simulink model "simulation_DICBF_"  (R2022a)
settings: Solver=VariableStepAuto  StartTime=0.0  StopTime=simTime  FixedStep=0.01  RelTol=1e-3
values from neighbouring files (symbols this model uses):
  Kd = 1    [setup.m]    (also in setup_DICBF.m)
  Kp = 0.2    [setup.m]    (also in setup_DICBF.m)
  M = 1*eye(2)    [setup.m]    (also in setup_DICBF.m)
  M2 = M    [setup_DICBF.m]
  mu = 1    [setup.m]    (also in setup_DICBF.m = 0.8)
  obstacles = setup_environment(MAP)    [setup_DICBF.m]
  qdotstart = [0,0]    [setup.m]    (also in setup_DICBF.m = [0 ; 0])
  qg = [4, -1]    [setup.m]    (also in setup_DICBF.m)
  qstart = [0,0]    [setup.m]    (also in setup_DICBF.m = [0 ; 0])
  threshold_skip = 0.0    (= 0)    [setup.m]    (also in setup_DICBF.m = 0.1)
libraries: slctrlblks x1
settings Model: Creator=mirkomizzoni  LastModifiedBy=dennis

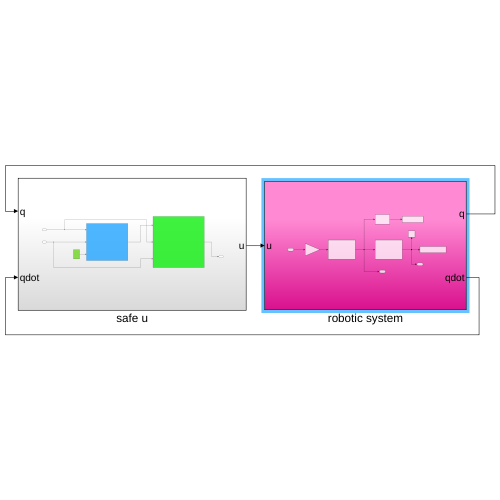
[thumbnail: Simulink's stored preview of the top-level diagram]
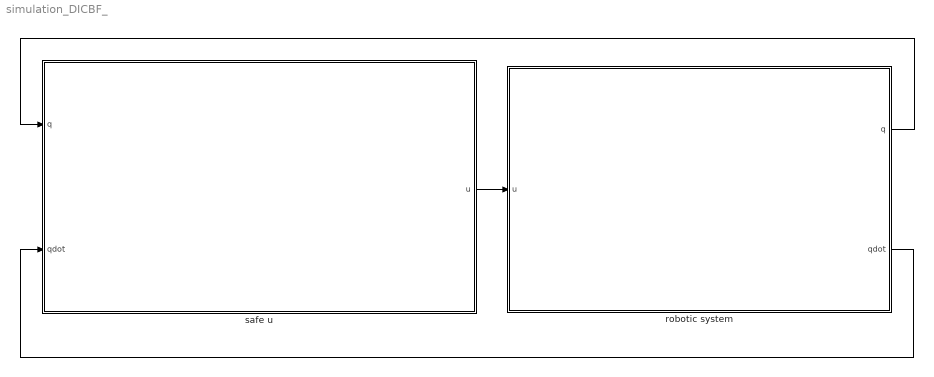
== system simulation_DICBF_ ==
  robotic system : Subsystem
  safe u : Subsystem
  wires:
  safe u/1(u) -> robotic system/1(u)
  robotic system/1(q) -> safe u/1(q)
  robotic system/2(qdot) -> safe u/2(qdot)

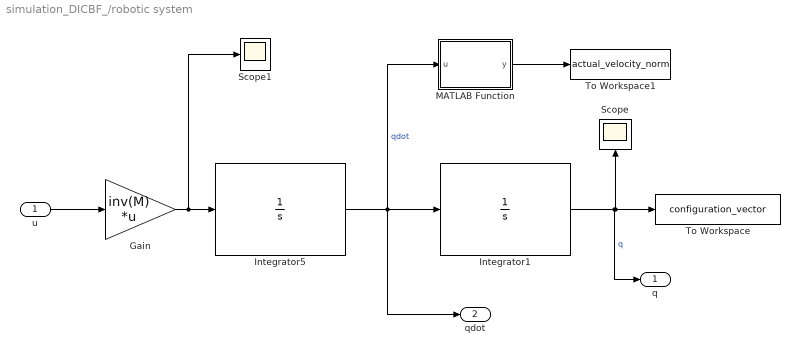
== system simulation_DICBF_/robotic system ==
  u : Inport
  Gain : Gain  Gain=inv(M)  Multiplication=Matrix(K*u)
  Integrator1 : Integrator  InitialCondition=qstart
  Integrator5 : Integrator  InitialCondition=qdotstart
  MATLAB Function : MATLAB Function  TreatAsAtomicUnit=on
  Scope : Scope
  Scope1 : Scope
  To Workspace : ToWorkspace  VariableName=configuration_vector  SaveFormat=Timeseries  SampleTime=0.01
  To Workspace1 : ToWorkspace  VariableName=actual_velocity_norm  SaveFormat=Timeseries  SampleTime=0.01
  q : Outport
  qdot : Outport  Port=2
  wires:
  Integrator5/1 -> qdot/1, MATLAB Function/1(u), Integrator1/1  "qdot"
  Integrator1/1 -> To Workspace/1, Scope/1, q/1  "q"
  MATLAB Function/1(y) -> To Workspace1/1
  Gain/1 -> Scope1/1, Integrator5/1
  u/1 -> Gain/1

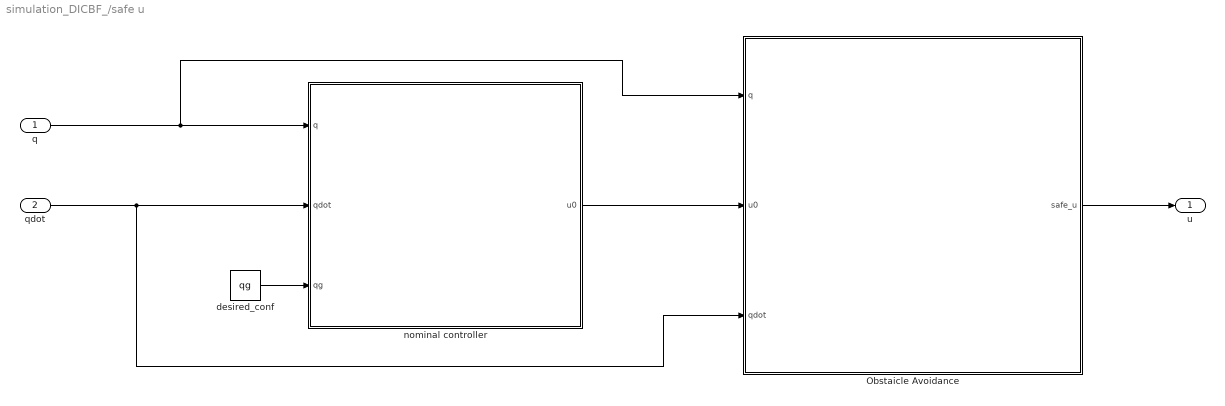
== system simulation_DICBF_/safe u ==
  q : Inport
  qdot : Inport  Port=2
  Obstaicle Avoidance : Subsystem
  desired_conf : Constant  Value=qg
  nominal controller : Subsystem
  u : Outport
  wires:
  desired_conf/1 -> nominal controller/3(qg)
  nominal controller/1(u0) -> Obstaicle Avoidance/2(u0)
  Obstaicle Avoidance/1(safe_u) -> u/1
  q/1 -> Obstaicle Avoidance/1(q), nominal controller/1(q)
  qdot/1 -> Obstaicle Avoidance/3(qdot), nominal controller/2(qdot)

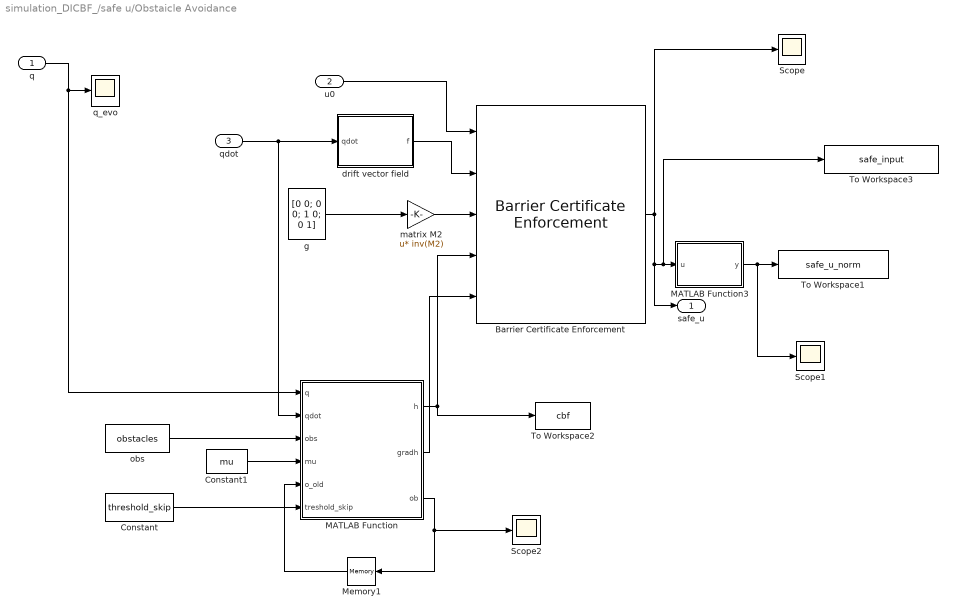
== system simulation_DICBF_/safe u/Obstaicle Avoidance ==
  q : Inport
  u0 : Inport  Port=2
  qdot : Inport  Port=3
  Barrier Certificate Enforcement : slctrlblks/Barrier Certificate Enforcement  nx=4  nu=2  nc=1  gamma=alpha  beta=1  external_umax=off  external_umin=off  Ts=0.01  maxiter=200  tol=1e-06  output_exitflag=off
      settings: SourceProductBaseCode=SD
  Constant : Constant  Value=threshold_skip
  Constant1 : Constant  Value=mu
  MATLAB Function : MATLAB Function  TreatAsAtomicUnit=on
  MATLAB Function3 : MATLAB Function  TreatAsAtomicUnit=on
  Memory1 : Memory  InitialCondition=obstacles(:,1);
  Scope : Scope
  Scope1 : Scope
  Scope2 : Scope
  To Workspace1 : ToWorkspace  VariableName=safe_u_norm  SaveFormat=Timeseries  SampleTime=0.01
  To Workspace2 : ToWorkspace  VariableName=cbf  SaveFormat=Timeseries  SampleTime=0.01
  To Workspace3 : ToWorkspace  VariableName=safe_input  SaveFormat=Timeseries  SampleTime=0.01
  drift vector field : MATLAB Function  TreatAsAtomicUnit=on
  g : Constant  Value=[0 0; 0 0; 1 0; 0 1]  VectorParams1D=off
  matrix M2 : Gain  Gain=inv(M2)  Multiplication=Matrix(u*K)
  obs : Constant  Value=obstacles  VectorParams1D=off
  q_evo : Scope
  safe_u : Outport
  wires:
  q/1 -> MATLAB Function/1(q), q_evo/1
  qdot/1 -> MATLAB Function/2(qdot), drift vector field/1(qdot)
  MATLAB Function3/1(y) -> Scope1/1, To Workspace1/1
  u0/1 -> Barrier Certificate Enforcement/1
  drift vector field/1(f) -> Barrier Certificate Enforcement/2
  Barrier Certificate Enforcement/1 -> To Workspace3/1, MATLAB Function3/1(u), safe_u/1, Scope/1
  g/1 -> matrix M2/1
  matrix M2/1 -> Barrier Certificate Enforcement/3
  MATLAB Function/1(h) -> Barrier Certificate Enforcement/4, To Workspace2/1
  Constant1/1 -> MATLAB Function/4(mu)
  obs/1 -> MATLAB Function/3(obs)
  Constant/1 -> MATLAB Function/6(treshold_skip)
  MATLAB Function/2(gradh) -> Barrier Certificate Enforcement/5
  MATLAB Function/3(ob) -> Scope2/1, Memory1/1
  Memory1/1 -> MATLAB Function/5(o_old)

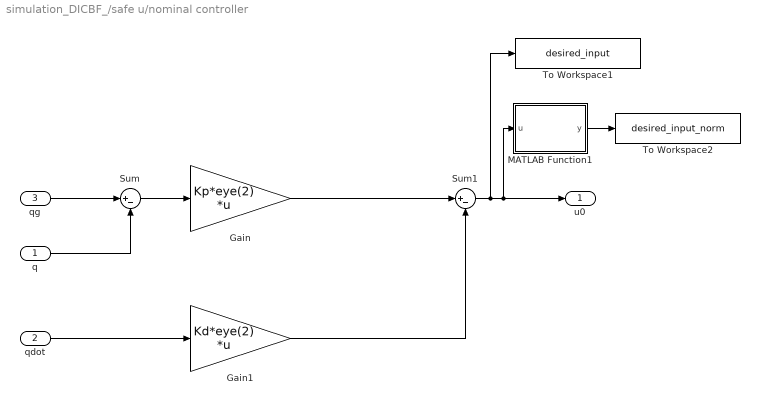
== system simulation_DICBF_/safe u/nominal controller ==
  q : Inport
  qdot : Inport  Port=2
  qg : Inport  Port=3
  Gain : Gain  Gain=Kp*eye(2)  Multiplication=Matrix(K*u)
  Gain1 : Gain  Gain=Kd*eye(2)  Multiplication=Matrix(K*u)
  MATLAB Function1 : MATLAB Function  TreatAsAtomicUnit=on
  Sum : Sum  Inputs=|+-
  Sum1 : Sum  Inputs=|+-
  To Workspace1 : ToWorkspace  VariableName=desired_input  SaveFormat=Timeseries  SampleTime=0.01
  To Workspace2 : ToWorkspace  VariableName=desired_input_norm  SaveFormat=Timeseries  SampleTime=0.01
  u0 : Outport
  wires:
  MATLAB Function1/1(y) -> To Workspace2/1
  q/1 -> Sum/2
  qg/1 -> Sum/1
  Sum/1 -> Gain/1
  Gain/1 -> Sum1/1
  qdot/1 -> Gain1/1
  Gain1/1 -> Sum1/2
  Sum1/1 -> To Workspace1/1, MATLAB Function1/1(u), u0/1

== matlab function simulation_DICBF_/safe u/Obstaicle Avoidance/MATLAB Function ==
  data: q input; qdot input; obs input; h output; gradh output; mu input; o_old input; treshold_skip input; ob output
function [h, gradh, ob]= compute_h_gradh(q, qdot, obs, mu, o_old, treshold_skip)
    [~,n] = size(obs);
    o1 = obs(:,1);
    h = first_part_h(q,o1)+second_part_h(o1(1:2),q,qdot,mu);
    gradh = gradient(o1(1:2),q, mu, qdot);
    ob = o1;
    for i=2:n
        oi = obs(:,i);
        t = first_part_h(q,oi)+second_part_h(oi(1:2),q,qdot,mu);
        if t<h
            h = t;
            gradh = gradient(oi(1:2),q, mu, qdot);
            ob = oi;
        end
    end
    h_old = first_part_h(q,o_old)+second_part_h(o_old(1:2),q,qdot,mu);
    if abs(h-h_old)<treshold_skip
        ob = o_old;
        h = h_old;
        gradh = gradient(ob(1:2),q, mu, qdot);
    end
end

function h1 = first_part_h(q, obs)
    h1 = norm(q-obs(1:2))-obs(3)-obs(4);
end

function h2 = second_part_h(qO,q,qdot, mu)
   h2 = mu*((q-qO)'*qdot);
end

function grad = gradient(qO,q, mu, qdot)
   gradp = 2*(q-qO)'+mu*qdot';
   grapdot = mu * (q-qO)';
   grad = [gradp, grapdot]; 
end

== matlab function simulation_DICBF_/robotic system/MATLAB Function ==
  data: u input; y output
function y = norm_func(u)
        
y = norm(u);

== matlab function simulation_DICBF_/safe u/Obstaicle Avoidance/MATLAB Function3 ==
  data: u input; y output
function y = norm_func(u)
        
y = norm(u);

== matlab function simulation_DICBF_/safe u/Obstaicle Avoidance/drift vector field ==
  data: qdot input; f output
function f = make_f(qdot)
    f = [qdot; 0; 0];
end

== matlab function simulation_DICBF_/safe u/nominal controller/MATLAB Function1 ==
  data: u input; y output
function y = norm_func(u)
        
y = norm(u);
